simulink model "Modelos"  (R2025a)
settings: Solver=FixedStepDiscrete  StartTime=0.0  StopTime=P.Tsim  FixedStep=P.Ts  RelTol=1e-3
InitFcn:
  | CarregaDados
values from neighbouring files (symbols this model uses):
  P = struct    [CarregaDados.m]
(part 2 of 2)

== matlab function Modelos/Task 01/Equações Modelo Discretizado/Função WAP ==
  data: W input; Ts input; Bypass input; ByPassWRC input; WAP output; P input
function WAP = fcn(W,Ts,Bypass,ByPassWRC,P)
    % Estados atuais
    WTD=W(1);  WQA=W(2);
    WRC=W(3);  WAP=W(4);

    % Extrai constantes dos parâmetros
    Ktd=P(1);     Kqa=P(2);      Krc=P(3);      Kap=P(4);
    Ptd=P(5);     Pqa=P(6);      Prc=P(7);      Pap=P(8);
    AlfaQA=P(9);  AlfaRC=P(10);  AlfaAP=P(11);

    % Entrada é a vazão de saida do tanque WRC, descontados os retrabalhos de RC
    Qin=(1-AlfaRC)*Krc*sqrt(WRC+Prc);  
 
    Qout=Kap*sqrt(WAP+Pap);  % Saida para avaliar trabalho aprovado ou retrabalho por não aprovação

    % Expressão da Eq.Diferencial
    Derivada = Qin - Qout;
    
    % Atualização do Estado
    WAP = WAP + Ts*Derivada;

    % Proteção, já que não faz sentido quantidades negativas para reciclos
    WAP=max(WAP,0);
end

== matlab function Modelos/Task 01/Equações Modelo Discretizado/Função WD ==
  data: W input; Ts input; WD output; P input
function WD = fcn(W,Ts,P)
    % Estados atuais
    WTD=W(1);  WQA=W(2);
    WRC=W(3);  WAP=W(4);
    WD=W(5);

    % Extrai constantes dos parâmetros
    Ktd=P(1);     Kqa=P(2);      Krc=P(3);      Kap=P(4);
    Ptd=P(5);     Pqa=P(6);      Prc=P(7);      Pap=P(8);
    AlfaQA=P(9);  AlfaRC=P(10);  AlfaAP=P(11);

    % Entrada é a vazão de saida do tanque WAP, descontados os retrabalhos de AP
    Qin=(1-AlfaAP)*Kap*sqrt(WAP+Pap);  

    % Saida =0
    Qout=0;

    % Expressão da Eq.Diferencial
    Derivada = Qin-Qout;    % Só acumula infinitamente o trabalho realizado
    
    % Atualização do Estado
    WD = WD + Ts*Derivada;

    % Proteção, já que não faz sentido quantidades negativas para reciclos
    WD=max(WD,0);
end

== matlab function Modelos/Task 01/Equações Modelo Discretizado/Função WQA ==
  data: W input; Ts input; Bypass input; WQA output; P input
function WQA = fcn(W,Ts,Bypass,P)
    % Estados atuais
    WTD=W(1);  WQA=W(2);
    WRC=W(3);  WAP=W(4);

    % Extrai constantes dos parâmetros
    Ktd=P(1);     Kqa=P(2);      Krc=P(3);      Kap=P(4);
    Ptd=P(5);     Pqa=P(6);      Prc=P(7);      Pap=P(8);
    AlfaQA=P(9);  AlfaRC=P(10);  AlfaAP=P(11);


    % Entrada é a vazão de saida do WTD
    Qin=Ktd*sqrt(WTD+Ptd);  

    Qout=Kqa*sqrt(WQA+Pqa);  % Saida para avaliar boa qualidade ou retrabalho

    % Expressão da Eq.Diferencial
    Derivada = Qin - Qout;
    
    % Atualização do Estado
    WQA = WQA + Ts*Derivada;

    % Proteção, já que não faz sentido quantidades negativas para reciclos
    WQA=max(WQA,0);
end

== matlab function Modelos/Task 01/Equações Modelo Discretizado/Função WRC ==
  data: W input; Ts input; Bypass input; BypassWQA input; WRC output; P input
function WRC = fcn(W,Ts,Bypass,BypassWQA,P)
    % Estados atuais
    WTD=W(1);  WQA=W(2);
    WRC=W(3);  WAP=W(4);

    % Extrai constantes dos parâmetros
    Ktd=P(1);     Kqa=P(2);      Krc=P(3);      Kap=P(4);
    Ptd=P(5);     Pqa=P(6);      Prc=P(7);      Pap=P(8);
    AlfaQA=P(9);  AlfaRC=P(10);  AlfaAP=P(11);

    % Entrada é a vazão de saida do tanque WQA, descontados os retrabalhos de QA
    Qin=(1-AlfaQA)*Kqa*sqrt(WQA+Pqa);  
    
    % Fluxo de saida de QRC
    Qout=Krc*sqrt(WRC+Prc);  % Saida para avaliar aprovação pelo cliente ou retrabalho

    % Expressão da Eq.Diferencial
    Derivada = Qin - Qout;
    
    % Atualização do Estado
    WRC = WRC + Ts*Derivada;

    % Proteção, já que não faz sentido quantidades negativas para reciclos
    WRC=max(WRC,0);
end

== matlab function Modelos/Task 01/Equações Modelo Discretizado/Função WTD ==
  data: KeepWaiting output; Waiting input; enable input; task_wu input; W input; Ts input; WTD output; P input
function [KeepWaiting,WTD] = fcn(Waiting,enable,task_wu,W,Ts,P)
    % Estados atuais
    WTD=W(1);  WQA=W(2);
    WRC=W(3);  WAP=W(4);

    if Waiting & enable & sum(W)==0 % Valeu só para condição incial
        WTD=task_wu;    % Força condição inicial igual ao WU da respectiva atividade
        KeepWaiting=0;  % Não precisa mais esperar
    else
        KeepWaiting=1;  % Continuar esperando o ENABLE
    end

    % Extrai constantes dos parâmetros
    Ktd=P(1);     Kqa=P(2);      Krc=P(3);      Kap=P(4);
    Ptd=P(5);     Pqa=P(6);      Prc=P(7);      Pap=P(8);
    AlfaQA=P(9);  AlfaRC=P(10);  AlfaAP=P(11);
    
    % Calcula as entradas por retrabalho
    ReQA=AlfaQA*Kqa*sqrt(WQA+Pqa);  % Por revisão interna
    ReRC=AlfaRC*Krc*sqrt(WRC+Prc);  % Por solicitação do cliente
    ReAP=AlfaAP*Kap*sqrt(WAP+Pap);  % Por não aprovação final
    ReWork=ReQA+ReRC+ReAP;          % Total de retrabalho

    % Expressão da Eq.Diferencial
    Derivada = 0 - Ktd*sqrt(WTD+Ptd) + ReWork;
    
    % Atualização do Estado
    WTD = WTD + Ts*Derivada;

    % Proteção, já que não faz sentido quantidades negativas para reciclos
    WTD=max(WTD,0);
end

== matlab function Modelos/Task 01/MATLAB Function ==
  data: enable input; Done output; Work input
function Done = fcn(enable,Work)
  
  if (enable) & (sum(Work(1:4))==0)   % Habilitado mas não tem mais nada para fazer
    Done = 1;  % Trabalho feito
  else
    Done = 0;  % Ainda há trabalho por fazer
  end
end

== matlab function Modelos/Task 06/Equações Modelo Discretizado/Função WAP ==
  data: x input; Ts input; WAP output; P input
function WAP = fcn(x,Ts,P)
    % Estados atuais
    WTD=x(1);  WQA=x(2);
    WRC=x(3);  WAP=x(4);

    % Extrai constantes dos parâmetros
    Ktd=P(1);     Kqa=P(2);      Krc=P(3);      Kap=P(4);
    Ptd=P(5);     Pqa=P(6);      Prc=P(7);      Pap=P(8);
    AlfaQA=P(9);  AlfaRC=P(10);  AlfaAP=P(11);

    % Entrada é a vazão de saida do tanque WRC, descontados os retrabalhos de RC
    Qin=(1-AlfaRC)*Krc*sqrt(WRC+Prc);  

    % Fluxo de saida de QAP
    Qout=Kap*sqrt(WAP+Pap);  % Saida para avaliar trabalho aprovado ou retrabalho por não aprovação

    % Expressão da Eq.Diferencial
    Derivada = Qin - Qout;
    
    % Atualização do Estado
    WAP = WAP + Ts*Derivada;

    % Proteção, já que não faz sentido quantidades negativas para reciclos
    WAP=max(WAP,0);
end

== matlab function Modelos/Task 06/Equações Modelo Discretizado/Função WD ==
  data: x input; Ts input; WD output; P input
function WD = fcn(x,Ts,P)
    % Estados atuais
    WTD=x(1);  WQA=x(2);
    WRC=x(3);  WAP=x(4);
    WD=x(5);

    % Extrai constantes dos parâmetros
    Ktd=P(1);     Kqa=P(2);      Krc=P(3);      Kap=P(4);
    Ptd=P(5);     Pqa=P(6);      Prc=P(7);      Pap=P(8);
    AlfaQA=P(9);  AlfaRC=P(10);  AlfaAP=P(11);

    % Entrada é a vazão de saida do tanque WAP, descontados os retrabalhos de AP
    Qin=(1-AlfaAP)*Kap*sqrt(WAP+Pap);  

    % Expressão da Eq.Diferencial
    Derivada = Qin;    % Só acumula infinitamente o trabalho realizado
    
    % Atualização do Estado
    WD = WD + Ts*Derivada;

    % Proteção, já que não faz sentido quantidades negativas para reciclos
    WD=max(WD,0);
end

== matlab function Modelos/Task 02/Equações Modelo Discretizado/Função WQA ==
  data: x input; Ts input; WQA output; P input
function WQA = fcn(x,Ts,P)
    % Estados atuais
    WTD=x(1);  WQA=x(2);
    WRC=x(3);  WAP=x(4);

    % Extrai constantes dos parâmetros
    Ktd=P(1);     Kqa=P(2);      Krc=P(3);      Kap=P(4);
    Ptd=P(5);     Pqa=P(6);      Prc=P(7);      Pap=P(8);
    AlfaQA=P(9);  AlfaRC=P(10);  AlfaAP=P(11);


    % Entrada é a vazão de saida do WTD
    Qin=Ktd*sqrt(WTD+Ptd);  

    % Fluxo de saida de QA
    Qout=Kqa*sqrt(WQA+Pqa);  % Saida para avaliar boa qualidade ou retrabalho

    % Expressão da Eq.Diferencial
    Derivada = Qin - Qout;
    
    % Atualização do Estado
    WQA = WQA + Ts*Derivada;

    % Proteção, já que não faz sentido quantidades negativas para reciclos
    WQA=max(WQA,0);
end

== matlab function Modelos/Task 06/Equações Modelo Discretizado/Função WQA ==
  data: x input; Ts input; WQA output; P input
function WQA = fcn(x,Ts,P)
    % Estados atuais
    WTD=x(1);  WQA=x(2);
    WRC=x(3);  WAP=x(4);

    % Extrai constantes dos parâmetros
    Ktd=P(1);     Kqa=P(2);      Krc=P(3);      Kap=P(4);
    Ptd=P(5);     Pqa=P(6);      Prc=P(7);      Pap=P(8);
    AlfaQA=P(9);  AlfaRC=P(10);  AlfaAP=P(11);


    % Entrada é a vazão de saida do WTD
    Qin=Ktd*sqrt(WTD+Ptd);  

    % Fluxo de saida de QA
    Qout=Kqa*sqrt(WQA+Pqa);  % Saida para avaliar boa qualidade ou retrabalho

    % Expressão da Eq.Diferencial
    Derivada = Qin - Qout;
    
    % Atualização do Estado
    WQA = WQA + Ts*Derivada;

    % Proteção, já que não faz sentido quantidades negativas para reciclos
    WQA=max(WQA,0);
end

== matlab function Modelos/Task 06/Equações Modelo Discretizado/Função WRC ==
  data: x input; Ts input; WRC output; P input
function WRC = fcn(x,Ts,P)
    % Estados atuais
    WTD=x(1);  WQA=x(2);
    WRC=x(3);  WAP=x(4);

    % Extrai constantes dos parâmetros
    Ktd=P(1);     Kqa=P(2);      Krc=P(3);      Kap=P(4);
    Ptd=P(5);     Pqa=P(6);      Prc=P(7);      Pap=P(8);
    AlfaQA=P(9);  AlfaRC=P(10);  AlfaAP=P(11);

    % Entrada é a vazão de saida do tanque WQA, descontados os retrabalhos de QA
    Qin=(1-AlfaQA)*Kqa*sqrt(WQA+Pqa);  

    % Fluxo de saida de QRC
    Qout=Krc*sqrt(WRC+Prc);  % Saida para avaliar aprovação pelo cliente ou retrabalho

    % Expressão da Eq.Diferencial
    Derivada = Qin - Qout;
    
    % Atualização do Estado
    WRC = WRC + Ts*Derivada;

    % Proteção, já que não faz sentido quantidades negativas para reciclos
    WRC=max(WRC,0);
end

== matlab function Modelos/Task 06/Equações Modelo Discretizado/Função WTD ==
  data: KeepWaiting output; Waiting input; enable input; task_wu input; x input; Ts input; WTD output; P input
function [KeepWaiting,WTD] = fcn(Waiting,enable,task_wu,x,Ts,P)
    % Estados atuais
    WTD=x(1);  WQA=x(2);
    WRC=x(3);  WAP=x(4);

    if Waiting & enable & sum(x)==0 % Valeu só para condição incial
        WTD=task_wu;    % Força condição inicial igual ao WU da respectiva atividade
        KeepWaiting=0;  % Não precisa mais esperar
    else
        KeepWaiting=1;  % Continuar esperando o ENABLE
    end

    % Extrai constantes dos parâmetros
    Ktd=P(1);     Kqa=P(2);      Krc=P(3);      Kap=P(4);
    Ptd=P(5);     Pqa=P(6);      Prc=P(7);      Pap=P(8);
    AlfaQA=P(9);  AlfaRC=P(10);  AlfaAP=P(11);
    
    % Calcula as entradas por retrabalho
    ReQA=AlfaQA*Kqa*sqrt(WQA+Pqa);  % Por revisão interna
    ReRC=AlfaRC*Krc*sqrt(WRC+Prc);  % Por solicitação do cliente
    ReAP=AlfaAP*Kap*sqrt(WAP+Pap);  % Por não aprovação final
    ReWork=ReQA+ReRC+ReAP;          % Total de retrabalho

    % Expressão da Eq.Diferencial
    Derivada = - Ktd*sqrt(WTD+Ptd) + ReWork;
    
    % Atualização do Estado
    WTD = WTD + Ts*Derivada;

    % Proteção, já que não faz sentido quantidades negativas para reciclos
    WTD=max(WTD,0);
end

== matlab function Modelos/Task 06/MATLAB Function ==
  data: enable input; Done output; Work input
function Done = fcn(enable,Work)
  
  if (enable) & (sum(Work(1:4))==0)   % Habilitado mas não tem mais nada para fazer
    Done = 1;  % Trabalho feito
  else
    Done = 0;  % Ainda há trabalho por fazer
  end
end

== matlab function Modelos/Task 07/Equações Modelo Discretizado/Função WAP ==
  data: x input; Ts input; WAP output; P input
function WAP = fcn(x,Ts,P)
    % Estados atuais
    WTD=x(1);  WQA=x(2);
    WRC=x(3);  WAP=x(4);

    % Extrai constantes dos parâmetros
    Ktd=P(1);     Kqa=P(2);      Krc=P(3);      Kap=P(4);
    Ptd=P(5);     Pqa=P(6);      Prc=P(7);      Pap=P(8);
    AlfaQA=P(9);  AlfaRC=P(10);  AlfaAP=P(11);

    % Entrada é a vazão de saida do tanque WRC, descontados os retrabalhos de RC
    Qin=(1-AlfaRC)*Krc*sqrt(WRC+Prc);  

    % Fluxo de saida de QAP
    Qout=Kap*sqrt(WAP+Pap);  % Saida para avaliar trabalho aprovado ou retrabalho por não aprovação

    % Expressão da Eq.Diferencial
    Derivada = Qin - Qout;
    
    % Atualização do Estado
    WAP = WAP + Ts*Derivada;

    % Proteção, já que não faz sentido quantidades negativas para reciclos
    WAP=max(WAP,0);
end

== matlab function Modelos/Task 07/Equações Modelo Discretizado/Função WD ==
  data: x input; Ts input; WD output; P input
function WD = fcn(x,Ts,P)
    % Estados atuais
    WTD=x(1);  WQA=x(2);
    WRC=x(3);  WAP=x(4);
    WD=x(5);

    % Extrai constantes dos parâmetros
    Ktd=P(1);     Kqa=P(2);      Krc=P(3);      Kap=P(4);
    Ptd=P(5);     Pqa=P(6);      Prc=P(7);      Pap=P(8);
    AlfaQA=P(9);  AlfaRC=P(10);  AlfaAP=P(11);

    % Entrada é a vazão de saida do tanque WAP, descontados os retrabalhos de AP
    Qin=(1-AlfaAP)*Kap*sqrt(WAP+Pap);  

    % Expressão da Eq.Diferencial
    Derivada = Qin;    % Só acumula infinitamente o trabalho realizado
    
    % Atualização do Estado
    WD = WD + Ts*Derivada;

    % Proteção, já que não faz sentido quantidades negativas para reciclos
    WD=max(WD,0);
end

== matlab function Modelos/Task 07/Equações Modelo Discretizado/Função WQA ==
  data: x input; Ts input; WQA output; P input
function WQA = fcn(x,Ts,P)
    % Estados atuais
    WTD=x(1);  WQA=x(2);
    WRC=x(3);  WAP=x(4);

    % Extrai constantes dos parâmetros
    Ktd=P(1);     Kqa=P(2);      Krc=P(3);      Kap=P(4);
    Ptd=P(5);     Pqa=P(6);      Prc=P(7);      Pap=P(8);
    AlfaQA=P(9);  AlfaRC=P(10);  AlfaAP=P(11);


    % Entrada é a vazão de saida do WTD
    Qin=Ktd*sqrt(WTD+Ptd);  

    % Fluxo de saida de QA
    Qout=Kqa*sqrt(WQA+Pqa);  % Saida para avaliar boa qualidade ou retrabalho

    % Expressão da Eq.Diferencial
    Derivada = Qin - Qout;
    
    % Atualização do Estado
    WQA = WQA + Ts*Derivada;

    % Proteção, já que não faz sentido quantidades negativas para reciclos
    WQA=max(WQA,0);
end

== matlab function Modelos/Task 07/Equações Modelo Discretizado/Função WRC ==
  data: x input; Ts input; WRC output; P input
function WRC = fcn(x,Ts,P)
    % Estados atuais
    WTD=x(1);  WQA=x(2);
    WRC=x(3);  WAP=x(4);

    % Extrai constantes dos parâmetros
    Ktd=P(1);     Kqa=P(2);      Krc=P(3);      Kap=P(4);
    Ptd=P(5);     Pqa=P(6);      Prc=P(7);      Pap=P(8);
    AlfaQA=P(9);  AlfaRC=P(10);  AlfaAP=P(11);

    % Entrada é a vazão de saida do tanque WQA, descontados os retrabalhos de QA
    Qin=(1-AlfaQA)*Kqa*sqrt(WQA+Pqa);  

    % Fluxo de saida de QRC
    Qout=Krc*sqrt(WRC+Prc);  % Saida para avaliar aprovação pelo cliente ou retrabalho

    % Expressão da Eq.Diferencial
    Derivada = Qin - Qout;
    
    % Atualização do Estado
    WRC = WRC + Ts*Derivada;

    % Proteção, já que não faz sentido quantidades negativas para reciclos
    WRC=max(WRC,0);
end

== matlab function Modelos/Task 07/Equações Modelo Discretizado/Função WTD ==
  data: KeepWaiting output; Waiting input; enable input; task_wu input; x input; Ts input; WTD output; P input
function [KeepWaiting,WTD] = fcn(Waiting,enable,task_wu,x,Ts,P)
    % Estados atuais
    WTD=x(1);  WQA=x(2);
    WRC=x(3);  WAP=x(4);

    if Waiting & enable & sum(x)==0 % Valeu só para condição incial
        WTD=task_wu;    % Força condição inicial igual ao WU da respectiva atividade
        KeepWaiting=0;  % Não precisa mais esperar
    else
        KeepWaiting=1;  % Continuar esperando o ENABLE
    end

    % Extrai constantes dos parâmetros
    Ktd=P(1);     Kqa=P(2);      Krc=P(3);      Kap=P(4);
    Ptd=P(5);     Pqa=P(6);      Prc=P(7);      Pap=P(8);
    AlfaQA=P(9);  AlfaRC=P(10);  AlfaAP=P(11);
    
    % Calcula as entradas por retrabalho
    ReQA=AlfaQA*Kqa*sqrt(WQA+Pqa);  % Por revisão interna
    ReRC=AlfaRC*Krc*sqrt(WRC+Prc);  % Por solicitação do cliente
    ReAP=AlfaAP*Kap*sqrt(WAP+Pap);  % Por não aprovação final
    ReWork=ReQA+ReRC+ReAP;          % Total de retrabalho

    % Expressão da Eq.Diferencial
    Derivada = - Ktd*sqrt(WTD+Ptd) + ReWork;
    
    % Atualização do Estado
    WTD = WTD + Ts*Derivada;

    % Proteção, já que não faz sentido quantidades negativas para reciclos
    WTD=max(WTD,0);
end

== matlab function Modelos/Task 02/Equações Modelo Discretizado/Função WRC ==
  data: x input; Ts input; WRC output; P input
function WRC = fcn(x,Ts,P)
    % Estados atuais
    WTD=x(1);  WQA=x(2);
    WRC=x(3);  WAP=x(4);

    % Extrai constantes dos parâmetros
    Ktd=P(1);     Kqa=P(2);      Krc=P(3);      Kap=P(4);
    Ptd=P(5);     Pqa=P(6);      Prc=P(7);      Pap=P(8);
    AlfaQA=P(9);  AlfaRC=P(10);  AlfaAP=P(11);

    % Entrada é a vazão de saida do tanque WQA, descontados os retrabalhos de QA
    Qin=(1-AlfaQA)*Kqa*sqrt(WQA+Pqa);  

    % Fluxo de saida de QRC
    Qout=Krc*sqrt(WRC+Prc);  % Saida para avaliar aprovação pelo cliente ou retrabalho

    % Expressão da Eq.Diferencial
    Derivada = Qin - Qout;
    
    % Atualização do Estado
    WRC = WRC + Ts*Derivada;

    % Proteção, já que não faz sentido quantidades negativas para reciclos
    WRC=max(WRC,0);
end

== matlab function Modelos/Task 07/MATLAB Function ==
  data: enable input; Done output; Work input
function Done = fcn(enable,Work)
  
  if (enable) & (sum(Work(1:4))==0)   % Habilitado mas não tem mais nada para fazer
    Done = 1;  % Trabalho feito
  else
    Done = 0;  % Ainda há trabalho por fazer
  end
end

== matlab function Modelos/Task Painel/MATLAB Function ==
  data: Enable input; Finished input; task_id input; Sel_Enable output; W input; Sel_Finished output; Sel_W output; Sum_W output
function [Sel_Enable,Sel_Finished,Sel_W,Sum_W] = fcn(Enable,Finished,task_id,W)
    W=reshape(W,5,7)';  % Reorganiza vetor de NumTafefas x 5 colunas 
    Sum_W=sum(W);       % Totaliza W em todas as atividades do projeto
    if task_id    % Foi selecionada uma atividade específica
        Sel_Enable=Enable(task_id);     % Enable da task selecionada
        Sel_Finished=Finished(task_id); % Finished da task selecionada
        Sel_W=W(task_id,:);
    else         % Para mostrar o resultado do projeto (todas as atividades)
        Sel_Enable=Enable(1);           % Todos os sinais de Enable
        Sel_Finished=Finished(end);     % Todos os sinais de Finished
        Sel_W=sum(W);                   % Totaliza W em todas as atividades do projeto
    end
end

== matlab function Modelos/Task Painel/MATLAB Function1 ==
  data: atual_W input; total_wu input; Wip output; Tr output
function [Wip,Tr] = fcn(atual_W,total_wu)
% Rotina para receber os diversos W e realizar algumas contas, gerando
% indices para análise do projeto

% Reorganiza vetor W em NumTarefas x 5 colunas
W=reshape(atual_W,5,7)';
W=sum(W);        % Totaliza as 5 colunas de W em todas as atividades do projeto
Wip=sum(W(1:4)); % Soma do que está em andamento (WTD+WQA+WRC+WAP)
Tr=Wip/total_wu; % Relação entre o que está feito e o que ainda tem por fazer

== matlab function Modelos/Task 02/Equações Modelo Discretizado/Função WTD ==
  data: KeepWaiting output; Waiting input; enable input; task_wu input; x input; Ts input; WTD output; P input
function [KeepWaiting,WTD] = fcn(Waiting,enable,task_wu,x,Ts,P)
    % Estados atuais
    WTD=x(1);  WQA=x(2);
    WRC=x(3);  WAP=x(4);

    if Waiting & enable & sum(x)==0 % Valeu só para condição incial
        WTD=task_wu;    % Força condição inicial igual ao WU da respectiva atividade
        KeepWaiting=0;  % Não precisa mais esperar
    else
        KeepWaiting=1;  % Continuar esperando o ENABLE
    end

    % Extrai constantes dos parâmetros
    Ktd=P(1);     Kqa=P(2);      Krc=P(3);      Kap=P(4);
    Ptd=P(5);     Pqa=P(6);      Prc=P(7);      Pap=P(8);
    AlfaQA=P(9);  AlfaRC=P(10);  AlfaAP=P(11);
    
    % Calcula as entradas por retrabalho
    ReQA=AlfaQA*Kqa*sqrt(WQA+Pqa);  % Por revisão interna
    ReRC=AlfaRC*Krc*sqrt(WRC+Prc);  % Por solicitação do cliente
    ReAP=AlfaAP*Kap*sqrt(WAP+Pap);  % Por não aprovação final
    ReWork=ReQA+ReRC+ReAP;          % Total de retrabalho

    % Expressão da Eq.Diferencial
    Derivada = - Ktd*sqrt(WTD+Ptd) + ReWork;
    
    % Atualização do Estado
    WTD = WTD + Ts*Derivada;

    % Proteção, já que não faz sentido quantidades negativas para reciclos
    WTD=max(WTD,0);
end

== matlab function Modelos/Task 02/MATLAB Function ==
  data: enable input; Done output; Work input
function Done = fcn(enable,Work)
  
  if (enable) & (sum(Work(1:4))==0)   % Habilitado mas não tem mais nada para fazer
    Done = 1;  % Trabalho feito
  else
    Done = 0;  % Ainda há trabalho por fazer
  end
end

== matlab function Modelos/Task 03/Equações Modelo Discretizado/Função WAP ==
  data: x input; Ts input; WAP output; P input
function WAP = fcn(x,Ts,P)
    % Estados atuais
    WTD=x(1);  WQA=x(2);
    WRC=x(3);  WAP=x(4);

    % Extrai constantes dos parâmetros
    Ktd=P(1);     Kqa=P(2);      Krc=P(3);      Kap=P(4);
    Ptd=P(5);     Pqa=P(6);      Prc=P(7);      Pap=P(8);
    AlfaQA=P(9);  AlfaRC=P(10);  AlfaAP=P(11);

    % Entrada é a vazão de saida do tanque WRC, descontados os retrabalhos de RC
    Qin=(1-AlfaRC)*Krc*sqrt(WRC+Prc);  

    % Fluxo de saida de QAP
    Qout=Kap*sqrt(WAP+Pap);  % Saida para avaliar trabalho aprovado ou retrabalho por não aprovação

    % Expressão da Eq.Diferencial
    Derivada = Qin - Qout;
    
    % Atualização do Estado
    WAP = WAP + Ts*Derivada;

    % Proteção, já que não faz sentido quantidades negativas para reciclos
    WAP=max(WAP,0);
end

== matlab function Modelos/Task 03/Equações Modelo Discretizado/Função WD ==
  data: x input; Ts input; WD output; P input
function WD = fcn(x,Ts,P)
    % Estados atuais
    WTD=x(1);  WQA=x(2);
    WRC=x(3);  WAP=x(4);
    WD=x(5);

    % Extrai constantes dos parâmetros
    Ktd=P(1);     Kqa=P(2);      Krc=P(3);      Kap=P(4);
    Ptd=P(5);     Pqa=P(6);      Prc=P(7);      Pap=P(8);
    AlfaQA=P(9);  AlfaRC=P(10);  AlfaAP=P(11);

    % Entrada é a vazão de saida do tanque WAP, descontados os retrabalhos de AP
    Qin=(1-AlfaAP)*Kap*sqrt(WAP+Pap);  

    % Expressão da Eq.Diferencial
    Derivada = Qin;    % Só acumula infinitamente o trabalho realizado
    
    % Atualização do Estado
    WD = WD + Ts*Derivada;

    % Proteção, já que não faz sentido quantidades negativas para reciclos
    WD=max(WD,0);
end

== matlab function Modelos/Task 03/Equações Modelo Discretizado/Função WQA ==
  data: x input; Ts input; WQA output; P input
function WQA = fcn(x,Ts,P)
    % Estados atuais
    WTD=x(1);  WQA=x(2);
    WRC=x(3);  WAP=x(4);

    % Extrai constantes dos parâmetros
    Ktd=P(1);     Kqa=P(2);      Krc=P(3);      Kap=P(4);
    Ptd=P(5);     Pqa=P(6);      Prc=P(7);      Pap=P(8);
    AlfaQA=P(9);  AlfaRC=P(10);  AlfaAP=P(11);


    % Entrada é a vazão de saida do WTD
    Qin=Ktd*sqrt(WTD+Ptd);  

    % Fluxo de saida de QA
    Qout=Kqa*sqrt(WQA+Pqa);  % Saida para avaliar boa qualidade ou retrabalho

    % Expressão da Eq.Diferencial
    Derivada = Qin - Qout;
    
    % Atualização do Estado
    WQA = WQA + Ts*Derivada;

    % Proteção, já que não faz sentido quantidades negativas para reciclos
    WQA=max(WQA,0);
end

== matlab function Modelos/Task 03/Equações Modelo Discretizado/Função WRC ==
  data: x input; Ts input; WRC output; P input
function WRC = fcn(x,Ts,P)
    % Estados atuais
    WTD=x(1);  WQA=x(2);
    WRC=x(3);  WAP=x(4);

    % Extrai constantes dos parâmetros
    Ktd=P(1);     Kqa=P(2);      Krc=P(3);      Kap=P(4);
    Ptd=P(5);     Pqa=P(6);      Prc=P(7);      Pap=P(8);
    AlfaQA=P(9);  AlfaRC=P(10);  AlfaAP=P(11);

    % Entrada é a vazão de saida do tanque WQA, descontados os retrabalhos de QA
    Qin=(1-AlfaQA)*Kqa*sqrt(WQA+Pqa);  

    % Fluxo de saida de QRC
    Qout=Krc*sqrt(WRC+Prc);  % Saida para avaliar aprovação pelo cliente ou retrabalho

    % Expressão da Eq.Diferencial
    Derivada = Qin - Qout;
    
    % Atualização do Estado
    WRC = WRC + Ts*Derivada;

    % Proteção, já que não faz sentido quantidades negativas para reciclos
    WRC=max(WRC,0);
end
